simulink model "analog_bp_4"  (Simulink 7.7)
settings: Solver=ode45  StartTime=0.0  StopTime=1  MaxStep=3e-6  RelTol=1e-3
values from neighbouring files (symbols this model uses):
  a = zeros(5, nord+1)    [analog_tp1.m]    (also in analog_tp2.m)
  b = fir1(nr-1,0.5)    [adapt_filter1.m]    (also in adapt_filter2.m; analog_tp1.m = zeros(5, nord+1); analog_tp2.m = zeros(5, nord+1))
libraries: commsynccomp2 x2
settings Model: Creator=svenhoffmann  LastModifiedBy=josef  ExtModeAutoUpdateStatusClock=off
settings DataIOCC: SignalLoggingName=sigsOut
settings DebuggingCC: SaveWithParameterizedLinksMsg=none  SignalResolutionControl=TryResolveAllWithWarning  SolverPrmCheckMsg=none  MultiTaskDSMMsg=warning  MultiTaskCondExecSysMsg=none  StrictBusMsg=None
settings HardwareCC: TargetUnknown=on
settings RTWCC: IncludeERTFirstTime=on

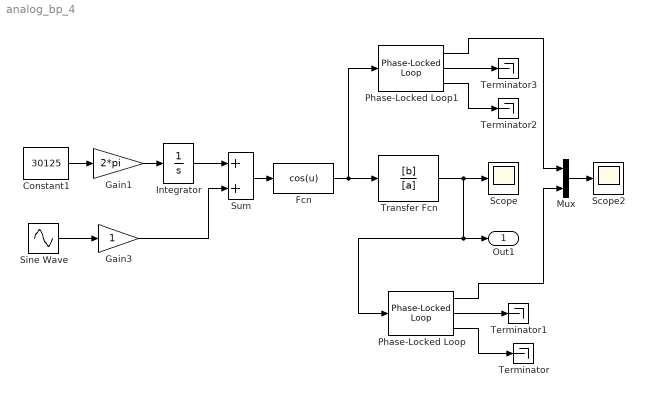
== system analog_bp_4 ==
  Constant1 : Constant  Value=30125
  Fcn : Fcn  Expr=cos(u)
  Gain1 : Gain  Gain=2*pi  SaturateOnIntegerOverflow=on  OutDataTypeStr=Inherit: Same as input  ParamDataTypeStr=Inherit: Same as input
  Gain3 : Gain  SaturateOnIntegerOverflow=on  OutDataTypeStr=Inherit: Same as input  ParamDataTypeStr=Inherit: Same as input
  Integrator : Integrator
  Mux : Mux  Inputs=2
  Phase-Locked Loop : commsynccomp2/Phase-Locked Loop  SystemSampleTime=-1  Fn=[1]  Fd=[1/2000 1]  Kvco=500  Fc=30125  Ph=0  Ac=1
  Phase-Locked Loop1 : commsynccomp2/Phase-Locked Loop  SystemSampleTime=-1  Fn=[1]  Fd=[1/2000 1]  Kvco=500  Fc=30125  Ph=0  Ac=1
  Scope : Scope
  Scope2 : Scope
      settings: YMin=-0.5  YMax=0.6  SaveName=ScopeData2
  Sine Wave : Sin  Frequency=2*pi*50  SampleTime=0
  Sum : Sum  SaturateOnIntegerOverflow=on
  Terminator{,1..3} (4 alike) : Terminator
  Transfer Fcn : TransferFcn  Numerator=[b]  Denominator=[a]
  Out1 : Outport
  wires:
  Fcn/1 -> Transfer Fcn/1, Phase-Locked Loop1/1
  Transfer Fcn/1 -> Scope/1, Out1/1, Phase-Locked Loop/1
  Sine Wave/1 -> Gain3/1
  Constant1/1 -> Gain1/1
  Gain1/1 -> Integrator/1
  Integrator/1 -> Sum/1
  Gain3/1 -> Sum/2
  Sum/1 -> Fcn/1
  Phase-Locked Loop/2 -> Terminator1/1
  Phase-Locked Loop/3 -> Terminator/1
  Phase-Locked Loop1/2 -> Terminator3/1
  Phase-Locked Loop1/3 -> Terminator2/1
  Phase-Locked Loop1/1 -> Mux/1
  Mux/1 -> Scope2/1
  Phase-Locked Loop/1 -> Mux/2
